simulink model "mathematic_functions"  (R2021a)
settings: Solver=FixedStepAuto  StartTime=-2*pi  StopTime=2*pi  FixedStep=pi/2000  RelTol=1e-3
settings Model: Creator=Acer  LastModifiedBy=Acer

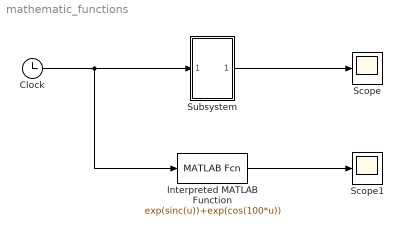
== system mathematic_functions ==
  Clock : Clock
  Interpreted MATLAB Function : MATLABFcn  MATLABFcn=exp(sinc(u))+exp(cos(100*u))  Output1D=off
  Scope : Scope
  Scope1 : Scope
  Subsystem : Subsystem
  wires:
  Clock/1 -> Interpreted MATLAB Function/1, Subsystem/1(In1)
  Subsystem/1(Out1) -> Scope/1
  Interpreted MATLAB Function/1 -> Scope1/1

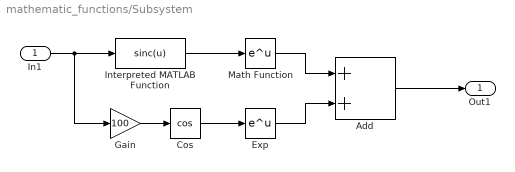
== system mathematic_functions/Subsystem ==
  In1 : Inport
  Add : Sum
  Cos : Trigonometry  Operator=cos
  Exp : Math  SaturateOnIntegerOverflow=on
  Gain : Gain  Gain=100
  Interpreted MATLAB Function : MATLABFcn  MATLABFcn=sinc(u)
  Math Function : Math  SaturateOnIntegerOverflow=on
  Out1 : Outport
  wires:
  Gain/1 -> Cos/1
  In1/1 -> Gain/1, Interpreted MATLAB Function/1
  Interpreted MATLAB Function/1 -> Math Function/1
  Cos/1 -> Exp/1
  Exp/1 -> Add/2
  Math Function/1 -> Add/1
  Add/1 -> Out1/1
